simulink model "sun_vs_nadir"  (R2021a)
settings: Solver=VariableStepAuto  StartTime=0.0  StopTime=7000  RelTol=1e-3
undefined symbols (not defined in the file or in its folder): dtheta_GMO, dtheta_LMO, I, i0_GMO, i0_LMO, K, Omega0_GMO, Omega0_LMO, P, r_GMO, r_LMO, T1, T2, theta0_GMO, theta0_LMO
libraries: sharedtransform x1
settings Model: Creator=VTX  LastModifiedBy=VTX

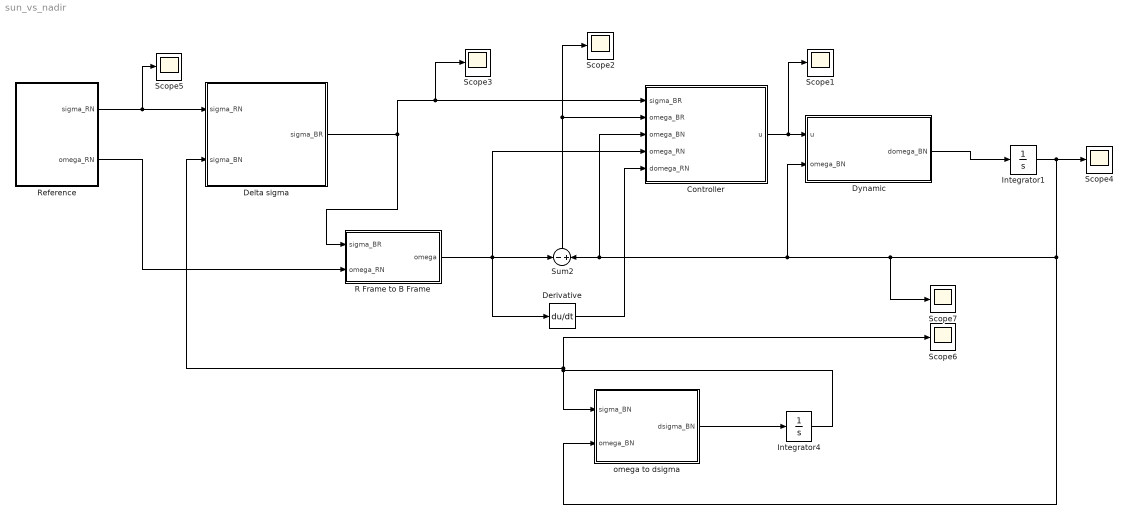
== system sun_vs_nadir ==
  Controller : MATLAB Function  TreatAsAtomicUnit=on
  Delta sigma : Subsystem
  Derivative : Derivative
  Dynamic : MATLAB Function  TreatAsAtomicUnit=on
  Integrator1 : Integrator  InitialCondition=[1;1.75;-2.2]*pi/180
  Integrator4 : Integrator  InitialCondition=[0.3;-0.4;0.5]
  R Frame to B Frame : MATLAB Function  TreatAsAtomicUnit=on
  Reference : Subsystem
  Scope{1..7} (7 alike) : Scope
  Sum2 : Sum  Inputs=-|+
  omega to dsigma : MATLAB Function  TreatAsAtomicUnit=on
  wires:
  Controller/1(u) -> Scope1/1, Dynamic/1(u)
  Delta sigma/1(sigma_BR) -> Scope3/1, Controller/1(sigma_BR), R Frame to B Frame/1(sigma_BR)
  omega to dsigma/1(dsigma_BN) -> Integrator4/1
  Reference/1(sigma_RN) -> Scope5/1, Delta sigma/1(sigma_RN)
  R Frame to B Frame/1(omega) -> Sum2/1, Derivative/1, Controller/4(omega_RN)
  Integrator1/1 -> Scope7/1, Dynamic/2(omega_BN), Controller/3(omega_BN), Sum2/2, omega to dsigma/2(omega_BN), Scope4/1
  Sum2/1 -> Scope2/1, Controller/2(omega_BR)
  Dynamic/1(domega_BN) -> Integrator1/1
  Reference/2(omega_RN) -> R Frame to B Frame/2(omega_RN)
  Derivative/1 -> Controller/5(domega_RN)
  Integrator4/1 -> Scope6/1, Delta sigma/2(sigma_BN), omega to dsigma/1(sigma_BN)

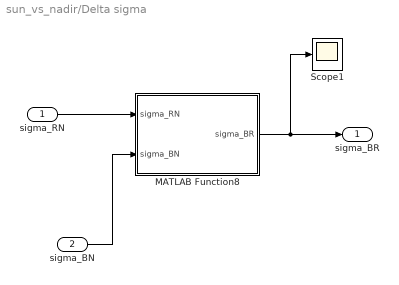
== system sun_vs_nadir/Delta sigma ==
  sigma_RN : Inport
  sigma_BN : Inport  Port=2
  MATLAB Function8 : MATLAB Function  TreatAsAtomicUnit=on
  Scope1 : Scope
  sigma_BR : Outport
  wires:
  sigma_BN/1 -> MATLAB Function8/2(sigma_BN)
  MATLAB Function8/1(sigma_BR) -> Scope1/1, sigma_BR/1
  sigma_RN/1 -> MATLAB Function8/1(sigma_RN)

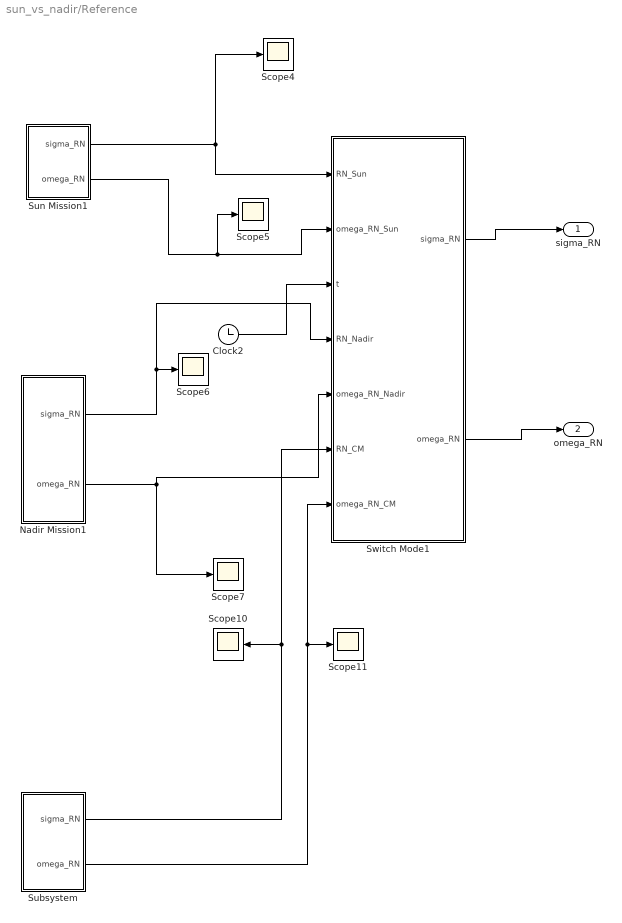
== system sun_vs_nadir/Reference ==
  Clock2 : Clock
  Nadir Mission1 : Subsystem
  Scope{4..7,10..11} (6 alike) : Scope
  Subsystem : Subsystem
  Sun Mission1 : Subsystem
  Switch Mode1 : MATLAB Function  TreatAsAtomicUnit=on
  sigma_RN : Outport
  omega_RN : Outport  Port=2
  wires:
  Switch Mode1/2(omega_RN) -> omega_RN/1
  Nadir Mission1/2(omega_RN) -> Scope7/1, Switch Mode1/5(omega_RN_Nadir)
  Switch Mode1/1(sigma_RN) -> sigma_RN/1
  Sun Mission1/1(sigma_RN) -> Scope4/1, Switch Mode1/1(RN_Sun)
  Clock2/1 -> Switch Mode1/3(t)
  Sun Mission1/2(omega_RN) -> Scope5/1, Switch Mode1/2(omega_RN_Sun)
  Nadir Mission1/1(sigma_RN) -> Scope6/1, Switch Mode1/4(RN_Nadir)
  Subsystem/1(sigma_RN) -> Scope10/1, Switch Mode1/6(RN_CM)
  Subsystem/2(omega_RN) -> Scope11/1, Switch Mode1/7(omega_RN_CM)

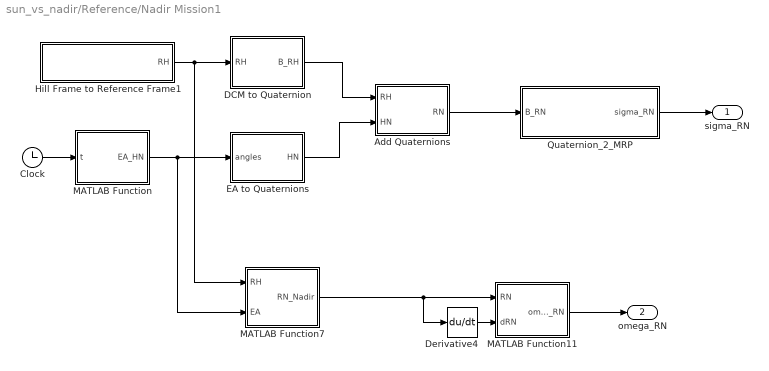
== system sun_vs_nadir/Reference/Nadir Mission1 ==
  Add Quaternions : MATLAB Function  TreatAsAtomicUnit=on
  Clock : Clock
  DCM to Quaternion : MATLAB Function  TreatAsAtomicUnit=on
  Derivative4 : Derivative
  EA to Quaternions : MATLAB Function  TreatAsAtomicUnit=on
  Hill Frame to Reference Frame1 : MATLAB Function  TreatAsAtomicUnit=on
  MATLAB Function : MATLAB Function  TreatAsAtomicUnit=on
  MATLAB Function11 : MATLAB Function  TreatAsAtomicUnit=on
  MATLAB Function7 : MATLAB Function  TreatAsAtomicUnit=on
  Quaternion_2_MRP : MATLAB Function  TreatAsAtomicUnit=on
  sigma_RN : Outport
  omega_RN : Outport  Port=2
  wires:
  Hill Frame to Reference Frame1/1(RH) -> MATLAB Function7/1(RH), DCM to Quaternion/1(RH)
  MATLAB Function/1(EA_HN) -> MATLAB Function7/2(EA), EA to Quaternions/1(angles)
  Clock/1 -> MATLAB Function/1(t)
  DCM to Quaternion/1(B_RH) -> Add Quaternions/1(RH)
  EA to Quaternions/1(HN) -> Add Quaternions/2(HN)
  Add Quaternions/1(RN) -> Quaternion_2_MRP/1(B_RN)
  Quaternion_2_MRP/1(sigma_RN) -> sigma_RN/1
  MATLAB Function7/1(RN_Nadir) -> Derivative4/1, MATLAB Function11/1(RN)
  Derivative4/1 -> MATLAB Function11/2(dRN)
  MATLAB Function11/1(omega_RN) -> omega_RN/1

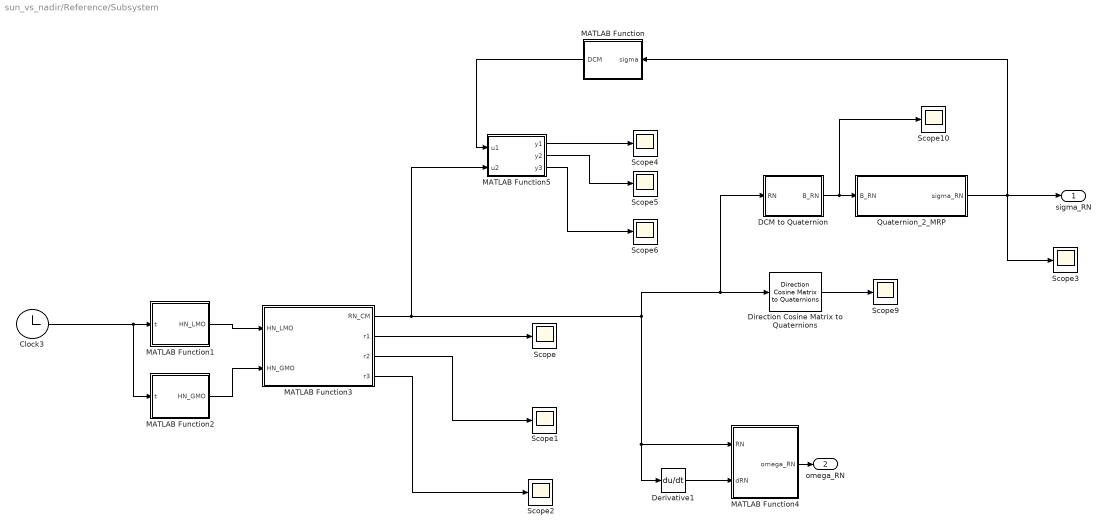
== system sun_vs_nadir/Reference/Subsystem ==
  Clock3 : Clock
  DCM to Quaternion : MATLAB Function  TreatAsAtomicUnit=on
  Derivative1 : Derivative
  Direction Cosine Matrix to Quaternions : sharedtransform/Direction Cosine Matrix  to Quaternions  aMode=0  action=None  tolerance=eps(2)
      settings: SourceProductBaseCode=AE,PW,DR,MT,UV,VE
  MATLAB Function : MATLAB Function  TreatAsAtomicUnit=on
  MATLAB Function1 : MATLAB Function  TreatAsAtomicUnit=on
  MATLAB Function2 : MATLAB Function  TreatAsAtomicUnit=on
  MATLAB Function3 : MATLAB Function  TreatAsAtomicUnit=on
  MATLAB Function4 : MATLAB Function  TreatAsAtomicUnit=on
  MATLAB Function5 : MATLAB Function  TreatAsAtomicUnit=on
  Quaternion_2_MRP : MATLAB Function  TreatAsAtomicUnit=on
  Scope{,1..6,9..10} (9 alike) : Scope
  sigma_RN : Outport
  omega_RN : Outport  Port=2
  wires:
  MATLAB Function2/1(HN_GMO) -> MATLAB Function3/2(HN_GMO)
  MATLAB Function4/1(omega_RN) -> omega_RN/1
  Direction Cosine Matrix to Quaternions/1 -> Scope9/1
  Clock3/1 -> MATLAB Function2/1(t), MATLAB Function1/1(t)
  MATLAB Function1/1(HN_LMO) -> MATLAB Function3/1(HN_LMO)
  Derivative1/1 -> MATLAB Function4/2(dRN)
  MATLAB Function3/1(RN_CM) -> MATLAB Function5/2(u2), Derivative1/1, MATLAB Function4/1(RN), DCM to Quaternion/1(RN), Direction Cosine Matrix to Quaternions/1
  DCM to Quaternion/1(B_RN) -> Scope10/1, Quaternion_2_MRP/1(B_RN)
  Quaternion_2_MRP/1(sigma_RN) -> MATLAB Function/1(sigma), Scope3/1, sigma_RN/1
  MATLAB Function3/2(r1) -> Scope/1
  MATLAB Function3/3(r2) -> Scope1/1
  MATLAB Function3/4(r3) -> Scope2/1
  MATLAB Function/1(DCM) -> MATLAB Function5/1(u1)
  MATLAB Function5/1(y1) -> Scope4/1
  MATLAB Function5/2(y2) -> Scope5/1
  MATLAB Function5/3(y3) -> Scope6/1

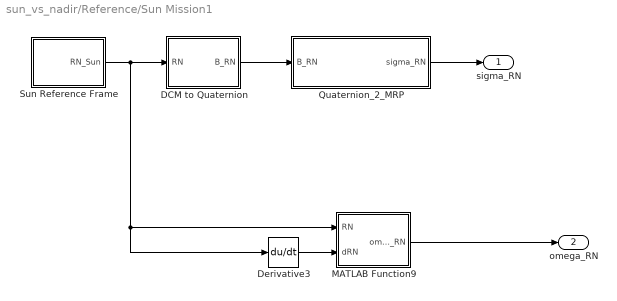
== system sun_vs_nadir/Reference/Sun Mission1 ==
  DCM to Quaternion : MATLAB Function  TreatAsAtomicUnit=on
  Derivative3 : Derivative
  MATLAB Function9 : MATLAB Function  TreatAsAtomicUnit=on
  Quaternion_2_MRP : MATLAB Function  TreatAsAtomicUnit=on
  Sun Reference Frame : MATLAB Function  TreatAsAtomicUnit=on
  sigma_RN : Outport
  omega_RN : Outport  Port=2
  wires:
  Derivative3/1 -> MATLAB Function9/2(dRN)
  MATLAB Function9/1(omega_RN) -> omega_RN/1
  Sun Reference Frame/1(RN_Sun) -> Derivative3/1, MATLAB Function9/1(RN), DCM to Quaternion/1(RN)
  DCM to Quaternion/1(B_RN) -> Quaternion_2_MRP/1(B_RN)
  Quaternion_2_MRP/1(sigma_RN) -> sigma_RN/1

== matlab function sun_vs_nadir/Reference/Nadir Mission1/Quaternion_2_MRP ==
  data: B_RN input; sigma_RN output
function sigma_RN  = fcn(B_RN)
    sigma1 = B_RN(2)/(1 + B_RN(1));
    sigma2 = B_RN(3)/(1 + B_RN(1));
    sigma3 = B_RN(4)/(1 + B_RN(1));
    
    sigma_RN = [sigma1 sigma2 sigma3]';
end

== matlab function sun_vs_nadir/Reference/Sun Mission1/DCM to Quaternion ==
  data: RN input; B_RN output size=4
function B_RN = fcn(RN)
    trace = RN(1,1) + RN(2,2) + RN(3,3);
    beta0 = (0.25*(1 + trace));
    beta1 = (0.25*(1 + 2*RN(1,1) - trace));
    beta2 = (0.25*(1 + 2*RN(2,2) - trace));
    beta3 = (0.25*(1 + 2*RN(3,3) - trace));
    
    m = max([beta0 beta1 beta2 beta3]);

    B0 = 0; B1 = 0; B2 = 0; B3 = 0;
    
    if beta0 == m
        B0 = sqrt(beta0);
        B1 = (RN(2,3)-RN(3,2))/(4*B0);
        B2 = (RN(3,1)-RN(1,3))/(4*B0);
        B3 = (RN(1,2)-RN(2,1))/(4*B0);
    elseif beta1 == m
        B1 = sqrt(beta1);
        B0 = (RN(2,3)-RN(3,2))/(4*B1);
        B2 = (RN(1,2)+RN(2,1))/(4*B1);
        B3 = (RN(3,1)+RN(1,3))/(4*B1);
    elseif beta2 == m
        B2 = sqrt(beta2);
        B0 = (RN(3,1)-RN(1,3))/(4*B2);
        B1 = (RN(1,2)+RN(2,1))/(4*B2);
        B3 = (RN(2,3)+RN(3,2))/(4*B2);
    elseif beta3 == m
        B3 = sqrt(beta3);
        B0 = (RN(1,2)-RN(2,1))/(4*B3);
        B1 = (RN(3,1)+RN(1,3))/(4*B3);
        B2 = (RN(2,3)+RN(3,2))/(4*B3);
    end
    
    B_RN = [B0 B1 B2 B3]';
end

== matlab function sun_vs_nadir/Reference/Sun Mission1/MATLAB Function9 ==
  data: RN input; omega_RN output; dRN input
function omega_RN = fcn(RN,dRN)
    omega_RN_tidle = -dRN*RN';
    o1 = omega_RN_tidle(3,2);
    o2 = omega_RN_tidle(1,3);
    o3 = omega_RN_tidle(2,1);
    omega_RN = [o1 o2 o3]';
end

== matlab function sun_vs_nadir/Reference/Sun Mission1/Quaternion_2_MRP ==
  data: B_RN input; sigma_RN output
function sigma_RN  = fcn(B_RN)
    sigma1 = B_RN(2)/(1 + B_RN(1));
    sigma2 = B_RN(3)/(1 + B_RN(1));
    sigma3 = B_RN(4)/(1 + B_RN(1));
    
    sigma_RN = [sigma1 sigma2 sigma3]';

    if norm(sigma_RN) >= 1
        sigma1 = -B_RN(2)/(1 - B_RN(1));
        sigma2 = -B_RN(3)/(1 - B_RN(1));
        sigma3 = -B_RN(4)/(1 - B_RN(1));
    
        sigma_RN = [sigma1 sigma2 sigma3]';
    end   
end

== matlab function sun_vs_nadir/Reference/Sun Mission1/Sun Reference Frame ==
  data: RN_Sun output
function RN_Sun = fcn()
    RN_Sun = [-1 0 0;0 0 1;0 1 0];
end

== matlab function sun_vs_nadir/Reference/Switch Mode1 ==
  data: RN_Sun input; omega_RN_Sun input; t input; RN_Nadir input; omega_RN_Nadir input; RN_CM input; omega_RN_CM input; sigma_RN output; omega_RN output; T1 parameter; T2 parameter
function [sigma_RN,omega_RN] = fcn(RN_Sun,omega_RN_Sun, t, RN_Nadir,omega_RN_Nadir,RN_CM,omega_RN_CM,T1, T2)
    sigma_RN = RN_CM;
    omega_RN = omega_RN_CM;
    
    if t > T1 && t <= T2
        sigma_RN = RN_Sun;
        omega_RN = omega_RN_Sun;
    elseif t > T2
        sigma_RN = RN_Nadir;
        omega_RN = omega_RN_Nadir;
    end
end

== matlab function sun_vs_nadir/Reference/Subsystem/MATLAB Function ==
  data: sigma input; DCM output
function DCM = MRP2DCM(sigma)
    %% This function returns a DCM that is transformed from MRP
    s1 = sigma(1);
    s2 = sigma(2);
    s3 = sigma(3);
    
    sigma_cross = [0 -s3 s2;s3 0 -s1;-s2 s1 0];
    
    DCM = eye(3) + (8*sigma_cross*sigma_cross - 4*(1 - dot(sigma,sigma))*sigma_cross)/(1 + dot(sigma,sigma))^2;

end

== matlab function sun_vs_nadir/Reference/Subsystem/MATLAB Function5 ==
  data: u1 input; u2 input; y1 output; y2 output; y3 output
function [y1,y2,y3] = fcn(u1,u2)
    y = u1 - u2;
    y1 = y(1,:);
    y2 = y(2,:);
    y3 = y(3,:);
end

== matlab function sun_vs_nadir/Reference/Subsystem/MATLAB Function1 ==
  data: t input; HN_LMO output; Omega0_LMO parameter; i0_LMO parameter; theta0_LMO parameter; dtheta_LMO parameter
function HN_LMO  = fcn(t,Omega0_LMO, i0_LMO, theta0_LMO, dtheta_LMO)
    %% Rotate about z axis
    Cz1 = [cos(Omega0_LMO) sin(Omega0_LMO) 0;-sin(Omega0_LMO) cos(Omega0_LMO) 0;0 0 1];

    %% Rotate about x axis
    Cx2 = [1 0 0;0 cos(i0_LMO) sin(i0_LMO);0 -sin(i0_LMO) cos(i0_LMO)];
    
    %% Rotate about z axis
    Cz3 = [cos(theta0_LMO + dtheta_LMO*t) sin(theta0_LMO + dtheta_LMO*t) 0;-sin(theta0_LMO + dtheta_LMO*t) cos(theta0_LMO + dtheta_LMO*t) 0;0 0 1];

    %% DCM from Inertial Frame to Hill Frame
    HN_LMO = Cz3*Cx2*Cz1;
end

== matlab function sun_vs_nadir/Reference/Subsystem/MATLAB Function2 ==
  data: t input; HN_GMO output; Omega0_GMO parameter; i0_GMO parameter; theta0_GMO parameter; dtheta_GMO parameter
function HN_GMO  = fcn(t,Omega0_GMO, i0_GMO, theta0_GMO, dtheta_GMO)
    %% Rotate about z axis
    Cz1 = [cos(Omega0_GMO) sin(Omega0_GMO) 0;-sin(Omega0_GMO) cos(Omega0_GMO) 0;0 0 1];

    %% Rotate about x axis
    Cx2 = [1 0 0;0 cos(i0_GMO) sin(i0_GMO);0 -sin(i0_GMO) cos(i0_GMO)];
    
    %% Rotate about z axis
    Cz3 = [cos(theta0_GMO + dtheta_GMO*t) sin(theta0_GMO + dtheta_GMO*t) 0;-sin(theta0_GMO + dtheta_GMO*t) cos(theta0_GMO + dtheta_GMO*t) 0;0 0 1];

    %% DCM from Inertial Frame to Hill Frame
    HN_GMO = Cz3*Cx2*Cz1;
end

== matlab function sun_vs_nadir/Reference/Nadir Mission1/Add Quaternions ==
  data: RH input; RN output; HN input
function RN = f(RH,HN)
    %% [BN] = [BR]*[RN]
    q0 = RH(1);
    q1 = RH(2);
    q2 = RH(3);
    q3 = RH(4);
    
    Matrix = [q0 -q1 -q2 -q3; ...
              q1 q0 q3 -q2; ...
              q2 -q3 q0 q1; ...
              q3 q2 -q1 q0];
    RN = Matrix*HN;
end

== matlab function sun_vs_nadir/Reference/Subsystem/MATLAB Function3 ==
  data: RN_CM output; HN_LMO input; HN_GMO input; r_LMO parameter; r_GMO parameter; r1 output; r2 output; r3 output
function [RN_CM,r1,r2,r3] = fcn(HN_LMO, HN_GMO,r_LMO, r_GMO)
    R_LMO = r_LMO*HN_LMO'*[1 0 0]';
    R_GMO = r_GMO*HN_GMO'*[1 0 0]';
    delta_R = R_GMO - R_LMO;
    
    r1 = delta_R/norm(delta_R);
    r2 = cross(delta_R,[0 0 1]')/norm(cross(delta_R,[0 0 1]'));
    r3 = cross(r1,r2);
    
    RN_CM = [r1 r2 r3]';
end

== matlab function sun_vs_nadir/Reference/Subsystem/MATLAB Function4 ==
  data: RN input; omega_RN output; dRN input
function omega_RN = fcn(RN,dRN)
    omega_RN_tidle = -dRN*RN';
    o1 = omega_RN_tidle(3,2);
    o2 = omega_RN_tidle(1,3);
    o3 = omega_RN_tidle(2,1);
    omega_RN = [o1 o2 o3]';
end

== matlab function sun_vs_nadir/Delta sigma/MATLAB Function8 ==
  data: sigma_BR output; sigma_RN input; sigma_BN input
function sigma_BR = fcn(sigma_RN, sigma_BN)
    sigma_BR = ((1 - norm(sigma_RN)^2)*sigma_BN - (1 - norm(sigma_BN)^2)*sigma_RN + 2*cross(sigma_BN,sigma_RN))/(1 + norm(sigma_RN)^2*norm(sigma_BN)^2 + 2*dot(sigma_RN,sigma_BN));
end

== matlab function sun_vs_nadir/Reference/Subsystem/DCM to Quaternion ==
  data: RN input; B_RN output size=4
function B_RN = fcn(RN)
    trace = RN(1,1) + RN(2,2) + RN(3,3);
    beta0 = (0.25*(1 + trace));
    beta1 = (0.25*(1 + 2*RN(1,1) - trace));
    beta2 = (0.25*(1 + 2*RN(2,2) - trace));
    beta3 = (0.25*(1 + 2*RN(3,3) - trace));
    
    m = max([beta0 beta1 beta2 beta3]);

    B0 = 0; B1 = 0; B2 = 0; B3 = 0;
    
    if beta0 == m
        B0 = sqrt(beta0);
        B1 = (RN(2,3)-RN(3,2))/(4*B0);
        B2 = (RN(3,1)-RN(1,3))/(4*B0);
        B3 = (RN(1,2)-RN(2,1))/(4*B0);
    elseif beta1 == m
        B1 = sqrt(beta1);
        B0 = (RN(2,3)-RN(3,2))/(4*B1);
        B2 = (RN(1,2)+RN(2,1))/(4*B1);
        B3 = (RN(3,1)+RN(1,3))/(4*B1);
    elseif beta2 == m
        B2 = sqrt(beta2);
        B0 = (RN(3,1)-RN(1,3))/(4*B2);
        B1 = (RN(1,2)+RN(2,1))/(4*B2);
        B3 = (RN(2,3)+RN(3,2))/(4*B2);
    elseif beta3 == m
        B3 = sqrt(beta3);
        B0 = (RN(1,2)-RN(2,1))/(4*B3);
        B1 = (RN(3,1)+RN(1,3))/(4*B3);
        B2 = (RN(2,3)+RN(3,2))/(4*B3);
    end
    
    B_RN = [B0 B1 B2 B3]';
end

== matlab function sun_vs_nadir/Reference/Subsystem/Quaternion_2_MRP ==
  data: B_RN input; sigma_RN output
function sigma_RN  = fcn(B_RN)
    sigma1 = B_RN(2)/(1 + B_RN(1));
    sigma2 = B_RN(3)/(1 + B_RN(1));
    sigma3 = B_RN(4)/(1 + B_RN(1));
    
    sigma_RN = [sigma1 sigma2 sigma3]';

    if norm(sigma_RN) >= 1
        sigma1 = -B_RN(2)/(1 - B_RN(1));
        sigma2 = -B_RN(3)/(1 - B_RN(1));
        sigma3 = -B_RN(4)/(1 - B_RN(1));
    
        sigma_RN = [sigma1 sigma2 sigma3]';
    end   
end

== matlab function sun_vs_nadir/omega to dsigma ==
  data: sigma_BN input; dsigma_BN output size=3; omega_BN input
function dsigma_BN = fcn(sigma_BN,omega_BN)
   sigma_tilde = [0 -sigma_BN(3) sigma_BN(2);sigma_BN(3) 0 -sigma_BN(1);-sigma_BN(2) sigma_BN(1) 0];
   dsigma_BN = 1/4*((1 - dot(sigma_BN,sigma_BN))*eye(3) + 2*sigma_tilde + 2*sigma_BN*sigma_BN')*omega_BN;
end

== matlab function sun_vs_nadir/Reference/Nadir Mission1/DCM to Quaternion ==
  data: RH input; B_RH output size=4
function B_RH = fcn(RH)
    trace = RH(1,1) + RH(2,2) + RH(3,3);
    beta0 = (0.25*(1 + trace));
    beta1 = (0.25*(1 + 2*RH(1,1) - trace));
    beta2 = (0.25*(1 + 2*RH(2,2) - trace));
    beta3 = (0.25*(1 + 2*RH(3,3) - trace));
    
    m = max([beta0 beta1 beta2 beta3]);

    B0 = 0; B1 = 0; B2 = 0; B3 = 0;
    
    if beta0 == m
        B0 = sqrt(beta0);
        B1 = (RH(2,3)-RH(3,2))/(4*B0);
        B2 = (RH(3,1)-RH(1,3))/(4*B0);
        B3 = (RH(1,2)-RH(2,1))/(4*B0);
    elseif beta1 == m
        B1 = sqrt(beta1);
        B0 = (RH(2,3)-RH(3,2))/(4*B1);
        B2 = (RH(1,2)+RH(2,1))/(4*B1);
        B3 = (RH(3,1)+RH(1,3))/(4*B1);
    elseif beta2 == m
        B2 = sqrt(beta2);
        B0 = (RH(3,1)-RH(1,3))/(4*B2);
        B1 = (RH(1,2)+RH(2,1))/(4*B2);
        B3 = (RH(2,3)+RH(3,2))/(4*B2);
    elseif beta3 == m
        B3 = sqrt(beta3);
        B0 = (RH(1,2)-RH(2,1))/(4*B3);
        B1 = (RH(3,1)+RH(1,3))/(4*B3);
        B2 = (RH(2,3)+RH(3,2))/(4*B3);
    end
    
    B_RH = [B0 B1 B2 B3]';
end

== matlab function sun_vs_nadir/Controller ==
  data: sigma_BR input; u output; omega_BR input; K parameter; P parameter; omega_BN input; omega_RN input; I parameter; domega_RN input
function u = fcn(sigma_BR,omega_BR,K,P,omega_BN,omega_RN, I,domega_RN)

    u = -K*sigma_BR - P*omega_BR;
    % u = -K*sigma_BR - P*omega_BR + I*(domega_RN - cross(omega_BN,omega_RN)) + cross(omega_BN,(I*omega_BN));
end

== matlab function sun_vs_nadir/Dynamic ==
  data: u input; domega_BN output size=3; omega_BN input; I parameter
function domega_BN = fcn(u,omega_BN, I)
    domega_BN = inv(I)*(-cross(omega_BN,(I*omega_BN)) + u);
end

== matlab function sun_vs_nadir/R Frame to B Frame ==
  data: omega output; sigma_BR input; omega_RN input
function omega = fcn(sigma_BR, omega_RN)
    %% This function returns a DCM that is transformed from MRP
    s1 = sigma_BR(1);
    s2 = sigma_BR(2);
    s3 = sigma_BR(3);
    
    sigma_cross = [0 -s3 s2;s3 0 -s1;-s2 s1 0];
    
    DCM = eye(3) + (8*sigma_cross*sigma_cross - 4*(1 - dot(sigma_BR,sigma_BR))*sigma_cross)/(1 + dot(sigma_BR,sigma_BR))^2;
    
    omega  = DCM*omega_RN;
end

== matlab function sun_vs_nadir/Reference/Nadir Mission1/EA to Quaternions ==
  data: angles input; HN output
function HN = EulerAngles313_2_Quaternions(angles)
    Omega = angles(1);
    i = angles(2);
    omega = angles(3);

    q0 = cos(omega/2)*cos(i/2)*cos(Omega/2) - sin(omega/2)*cos(i/2)*sin(Omega/2);
    q1 = cos(omega/2)*sin(i/2)*cos(Omega/2) + sin(omega/2)*sin(i/2)*sin(Omega/2);
    q2 = -sin(omega/2)*sin(i/2)*cos(Omega/2) + cos(omega/2)*sin(i/2)*sin(Omega/2);
    q3 = sin(omega/2)*cos(i/2)*cos(Omega/2) + cos(omega/2)*cos(i/2)*sin(Omega/2);
    
    HN = [q0 q1 q2 q3]';
end

== matlab function sun_vs_nadir/Reference/Nadir Mission1/Hill Frame to Reference Frame1 ==
  data: RH output
function RH = fcn()
RH = [-1 0 0;0 1 0;0 0 -1];
end

== matlab function sun_vs_nadir/Reference/Nadir Mission1/MATLAB Function ==
  data: t input; EA_HN output; Omega0_LMO parameter; i0_LMO parameter; theta0_LMO parameter; dtheta_LMO parameter
function EA_HN = fcn(t,Omega0_LMO, i0_LMO, theta0_LMO, dtheta_LMO)
    EA_HN = [Omega0_LMO i0_LMO (theta0_LMO + dtheta_LMO*t)]';
end

== matlab function sun_vs_nadir/Reference/Nadir Mission1/MATLAB Function11 ==
  data: RN input; omega_RN output; dRN input
function omega_RN = fcn(RN,dRN)
    omega_RN_tidle = -dRN*RN';
    o1 = omega_RN_tidle(3,2);
    o2 = omega_RN_tidle(1,3);
    o3 = omega_RN_tidle(2,1);
    omega_RN = [o1 o2 o3]';
end

== matlab function sun_vs_nadir/Reference/Nadir Mission1/MATLAB Function7 ==
  data: RN_Nadir output; RH input; EA input
function RN_Nadir  = fcn(RH,EA)
    Omega = EA(1);
    i = EA(2);
    theta = EA(3);

    %% Rotate about z axis
    Cz1 = [cos(Omega) sin(Omega) 0;-sin(Omega) cos(Omega) 0;0 0 1];

    %% Rotate about x axis
    Cx2 = [1 0 0;0 cos(i) sin(i);0 -sin(i) cos(i)];
    
    %% Rotate about z axis
    Cz3 = [cos(theta) sin(theta) 0;-sin(theta) cos(theta) 0;0 0 1];

    %% DCM from Inertial Frame to Hill Frame
    HN = Cz3*Cx2*Cz1;
    
    %% DCm from Inertial Frame to Reference Frame
    RN_Nadir = RH*HN;
end
